simulink model "bulk_boost_eq"  (R2020b)
settings: Solver=VariableStepAuto  StartTime=0.0  StopTime=0.6  FixedStep=t_step
undefined symbols (not defined in the file): Cb, ki_1, kp_1, Lb, Rb, t_step, Vc, Vl, Vs
libraries: powerlib x18, powerlib_meascontrol x1
settings Model: Creator=Chuanyue Li  LastModifiedBy=kjaku
settings DataIOCC: ReturnWorkspaceOutputs=off
settings DebuggingCC: ArithmeticOperatorsInVariantConditions=warning
settings SFSimCC: SimUseLocalCustomCode=off  CustomCodeUndefinedFunction=UseInterfaceOnly
settings RTWCC: RTWUseLocalCustomCode=off

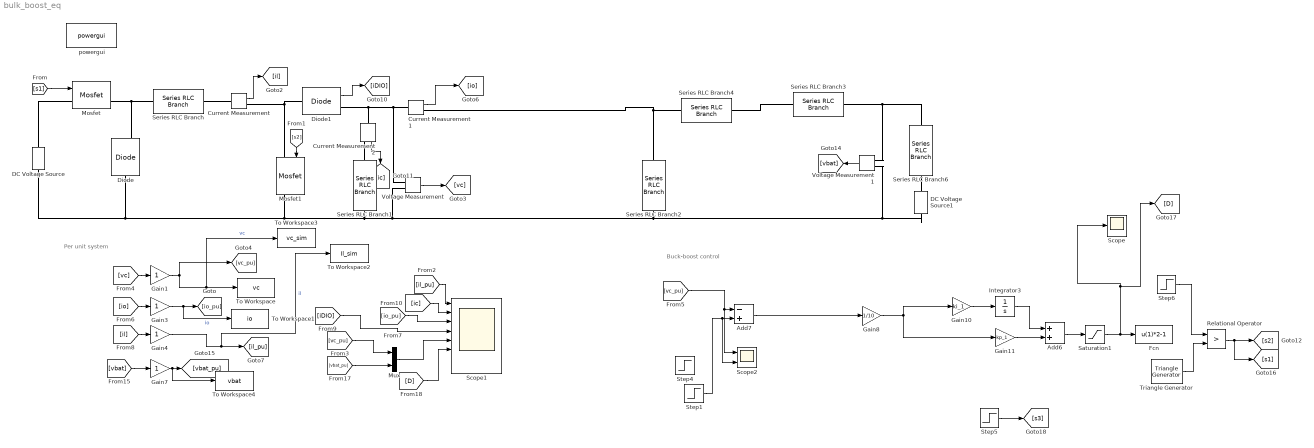
== system bulk_boost_eq ==
  note: Per unit system
  note: Buck-boost control
  Add6 : Sum
  Add7 : Sum  Inputs=-+
  Current Measurement : powerlib/Measurements/Current Measurement  PhasorSimulation=off  OutputType=Complex  PSBequivalent=0
  Current Measurement1 : powerlib/Measurements/Current Measurement  PhasorSimulation=off  OutputType=Complex  PSBequivalent=0
  Current Measurement2 : powerlib/Measurements/Current Measurement  PhasorSimulation=off  OutputType=Complex  PSBequivalent=0
  DC Voltage Source : powerlib/Electrical Sources/DC Voltage Source  Amplitude=Vs  Measurements=None
  DC Voltage Source1 : powerlib/Electrical Sources/DC Voltage Source  Amplitude=Vl  Measurements=None
  Diode : powerlib/Power Electronics/Diode  Ron=0.001  Lon=0  Vf=0  IC=0  UseSnubber=0  Rs=500000  Cs=250e-9  Measurements=on
  Diode1 : powerlib/Power Electronics/Diode  Ron=0.001  Lon=0  Vf=0  IC=0  UseSnubber=0  Rs=500000  Cs=250e-9  Measurements=on
  Fcn : Fcn  Expr=u(1)*2-1
  Gain{1,3..4,7} (4 alike) : Gain
  Gain10 : Gain  Gain=ki_1
  Gain11 : Gain  Gain=kp_1
  Gain8 : Gain  Gain=1/10
  Integrator3 : Integrator  InitialCondition=0.7
  Mosfet : powerlib/Power Electronics/Mosfet  Ron=0.01  Lon=0  Rd=0.01  Vfd=0  IC=0  Rs=1e5  Cs=inf  Measurements=on
  Mosfet1 : powerlib/Power Electronics/Mosfet  Ron=0.01  Lon=0  Rd=0.01  Vfd=0  IC=0  Rs=1e5  Cs=inf  Measurements=on
  Mux : Mux  Inputs=2
  Relational Operator : RelationalOperator  Operator=>  OutDataTypeStr=boolean  RndMeth=Zero
  Saturation1 : Saturate  UpperLimit=0.95  LowerLimit=-0.95
  Scope : Scope
  Scope1 : Scope  NumInputPorts=8
  Scope2 : Scope  NumInputPorts=2
  Series RLC Branch : powerlib/Elements/Series RLC Branch  LConnTagsString=__new0  RConnTagsString=__new0  BranchType=L  Resistance=1  Inductance=Lb  SetiL0=off  InitialCurrent=0  Capacitance=1e-6  Setx0=off  InitialVoltage=0  Measurements=None
  Series RLC Branch1 : powerlib/Elements/Series RLC Branch  LConnTagsString=__new0  RConnTagsString=__new0  BranchType=C  Resistance=1  Inductance=1e-3  SetiL0=off  InitialCurrent=0  Capacitance=Cb  Setx0=off  InitialVoltage=0  Measurements=None
  Series RLC Branch2 : powerlib/Elements/Series RLC Branch  LConnTagsString=__new0  RConnTagsString=__new0  BranchType=C  Resistance=1  Inductance=1e-3  SetiL0=off  InitialCurrent=0  Capacitance=Cb/1.9/1.3  Setx0=off  InitialVoltage=0  Measurements=None
  Series RLC Branch3 : powerlib/Elements/Series RLC Branch  LConnTagsString=__new0  RConnTagsString=__new0  BranchType=R  Resistance=Rb*100  Inductance=Lb  SetiL0=off  InitialCurrent=0  Capacitance=1e-6  Setx0=off  InitialVoltage=0  Measurements=None
  Series RLC Branch4 : powerlib/Elements/Series RLC Branch  LConnTagsString=__new0  RConnTagsString=__new0  BranchType=L  Resistance=1  Inductance=Lb*100*1.3  SetiL0=off  InitialCurrent=0  Capacitance=1e-6  Setx0=off  InitialVoltage=0  Measurements=None
  Series RLC Branch6 : powerlib/Elements/Series RLC Branch  LConnTagsString=__new0  RConnTagsString=__new0  BranchType=R  Resistance=Rb  Inductance=Lb  SetiL0=off  InitialCurrent=0  Capacitance=1e-6  Setx0=off  InitialVoltage=0  Measurements=None
  Step1 : Step  Time=0.4  Before=Vc  After=Vc*1.1  SampleTime=0
  Step4 : Step  Time=0.4  Before=Vc  After=Vc+5  SampleTime=0
  Step5 : Step  Time=0.05  Before=1  SampleTime=0
  Step6 : Step  Time=0.3  Before=0.55  After=0.6  SampleTime=0
  To Workspace : ToWorkspace  VariableName=vc  SaveFormat=Timeseries  SampleTime=-1
  To Workspace1 : ToWorkspace  VariableName=io  SaveFormat=Timeseries  SampleTime=-1
  To Workspace2 : ToWorkspace  VariableName=Il_sim  SaveFormat=Timeseries  SampleTime=-1
  To Workspace3 : ToWorkspace  VariableName=vc_sim  SaveFormat=Timeseries  SampleTime=-1
  To Workspace4 : ToWorkspace  VariableName=vbat  SaveFormat=Timeseries  SampleTime=-1
  Triangle Generator : powerlib_meascontrol/Pulse & Signal Generators/Triangle Generator  Freq=s_fre  Phase=0  Ts=0
  Voltage Measurement : powerlib/Measurements/Voltage Measurement  PhasorSimulation=off  OutputType=Complex  PSBequivalent=0
  Voltage Measurement1 : powerlib/Measurements/Voltage Measurement  PhasorSimulation=off  OutputType=Complex  PSBequivalent=0
  powergui : powerlib/powergui  Priority=1  SimulationMode=Continuous  SampleTime=t_step  frequency=60  Iterations=50  frequencyindice=0  Pbase=100e6  ErrMax=1e-4  UnitsV=kV  UnitsW=MW  buscounter=0  FunctionMessages=off  echomessages=off  EnableUseOfTLC=off  CurrentSourceSwitches=off  DisableSnubberDevices=off  DisableRonSwitches=off  DisableVfSwitches=off  DisplayEquations=off  AutomaticDiscreteSolvers=off  SolverType=Tustin/Backward Euler (TBE)  Interpol=off  ExternalGateDelay=off  methode=off  Ts=100  x0status=blocks  SPID=off  SwTol=0  HookPort=off  NonlinearTolerance=1e-4  nMaxIteration=100  ContinueOnMaxIteration=off  RestoreLinks=warning  ResistiveCurrentMeasurement=off  Frange=[0:2:500]  Ylog=off  Xlog=on  ShowGrid=off  save=off  variable=ZData  structure=logsout  ZoomFFT=off  StartTime=0.2  cycles=10  DisplayStyle=2  fundamental=50  FreqAxis=off  MaxFrequency=1000  frequencyindicesteady=1  RmsSteady=1  display=off
  wires:
  [s1] -> Mosfet/1
  [s2] -> Mosfet1/1
  Current Measurement/1 -> [il]
  Voltage Measurement/1 -> [vc]
  [il_pu] -> Scope1/1
  [vc] -> Gain1/1
  Gain1/1 -> To Workspace3/1, To Workspace/1, [vc_pu]  "vc"
  [io] -> Gain3/1
  Current Measurement1/1 -> [io]
  Gain3/1 -> To Workspace1/1, [io_pu]  "io"
  [io_pu] -> Scope1/3
  Gain4/1 -> To Workspace2/1, [il_pu]  "il"
  [il] -> Gain4/1
  Diode1/1 -> [iDIO]
  [iDIO] -> Scope1/4
  Current Measurement2/1 -> [ic]
  [ic] -> Scope1/2
  Voltage Measurement1/1 -> [vbat]
  [vbat] -> Gain7/1
  Gain7/1 -> To Workspace4/1, [vbat_pu]
  [vc_pu] -> Mux/1
  Mux/1 -> Scope1/5
  [vbat_pu] -> Mux/2
  Triangle Generator/1 -> Relational Operator/2
  Step6/1 -> Relational Operator/1
  Relational Operator/1 -> [s1], [s2]
  Step5/1 -> [s3]
  Add6/1 -> Saturation1/1
  Integrator3/1 -> Add6/1
  Gain11/1 -> Add6/2
  Saturation1/1 -> [D], Scope/1, Fcn/1
  [vc_pu] -> Scope2/1, Add7/1
  Gain10/1 -> Integrator3/1
  Gain8/1 -> Gain11/1, Gain10/1
  Step1/1 -> Scope2/2, Add7/2
  [D] -> Scope1/6
  Add7/1 -> Gain8/1
  connections:
  DC Voltage Source/RConn1 -- Mosfet/LConn1
  Mosfet/RConn1 -- Diode/RConn1 -- Series RLC Branch/LConn1
  Mosfet1/LConn1 -- Current Measurement/RConn1 -- Diode1/LConn1
  Diode/LConn1 -- DC Voltage Source/LConn1 -- Voltage Measurement1/LConn2 -- DC Voltage Source1/LConn1 -- Series RLC Branch2/RConn1 -- Voltage Measurement/LConn2 -- Series RLC Branch1/RConn1 -- Mosfet1/RConn1
  Current Measurement1/LConn1 -- Voltage Measurement/LConn1 -- Current Measurement2/LConn1 -- Diode1/RConn1
  Current Measurement/LConn1 -- Series RLC Branch/RConn1
  Current Measurement2/RConn1 -- Series RLC Branch1/LConn1
  Series RLC Branch3/LConn1 -- Voltage Measurement1/LConn1 -- Series RLC Branch6/RConn1
  Series RLC Branch2/LConn1 -- Series RLC Branch4/RConn1 -- Current Measurement1/RConn1
  Series RLC Branch6/LConn1 -- DC Voltage Source1/RConn1
  Series RLC Branch4/LConn1 -- Series RLC Branch3/RConn1
